simulink model "frbd_64ch_600mhz"  (R2013b)
settings: Solver=FixedStepDiscrete  SolverMode=SingleTasking  StartTime=0.0  StopTime=10.0  RelTol=1e-3
undefined symbols (not defined in the file or in its folder): pfb_coeff_gen_calc
libraries: xbsIndex_r4 x14695, casper_library_misc x59, casper_library_delays x32, dspsigops x16, casper_library_pfbs x2, xps_library x1
(part 24 of 145)

== system frbd_64ch_600mhz/Parallel_Dedispersor_v4/Dedispersor_v2_4 ==
  Data : Inport
  Valid : Inport  Port=2
  Counter : xbsIndex_r4/Counter  cnt_type=Free Running  cnt_to=Inf  operation=Up  start_count=0  cnt_by_val=1  arith_type=Unsigned  n_bits=4  bin_pt=0  load_pin=off  rst=off  en=on  explicit_period=on  period=1  dbl_ovrd=off  use_behavioral_HDL=off  implementation=Fabric  block_type=counter
  Mux : xbsIndex_r4/Mux  inputs=16  en=off  latency=0  precision=Full  arith_type=Unsigned  n_bits=16  bin_pt=14  quantization=Truncate  overflow=Wrap  dbl_ovrd=off  block_type=mux
  detector_block_v2 : Subsystem  AncestorBlock=honestlibrary/detector_block_v2  mask(Basic block for FRB detection){chn=0, lat=8, nbits=4}
      mask prompts: chn "Channel"; lat "Latency"; nbits "Number of Bits (Counter)"
      mask help:
      | Delays a certain channel a number of latency clock cycles, according to the fixed DM table.
      | This version incorporates an internal counter (nbits) to know when store or give a certain value.
      mask init:
      | detector_block_init_v2(gcb,'chn',chn,'lat',lat,'nbits',nbits)
      settings: AttributesFormatString=Channel: 0, Delay: 8
  detector_block_v21 : Subsystem  AncestorBlock=honestlibrary/detector_block_v2  mask(Basic block for FRB detection){chn=1, lat=20, nbits=4}
      mask prompts: chn "Channel"; lat "Latency"; nbits "Number of Bits (Counter)"
      mask help:
      | Delays a certain channel a number of latency clock cycles, according to the fixed DM table.
      | This version incorporates an internal counter (nbits) to know when store or give a certain value.
      mask init:
      | detector_block_init_v2(gcb,'chn',chn,'lat',lat,'nbits',nbits)
      settings: AttributesFormatString=Channel: 1, Delay: 20
  detector_block_v210 : Subsystem  AncestorBlock=honestlibrary/detector_block_v2  mask(Basic block for FRB detection){chn=10, lat=93, nbits=4}
      mask prompts: chn "Channel"; lat "Latency"; nbits "Number of Bits (Counter)"
      mask help:
      | Delays a certain channel a number of latency clock cycles, according to the fixed DM table.
      | This version incorporates an internal counter (nbits) to know when store or give a certain value.
      mask init:
      | detector_block_init_v2(gcb,'chn',chn,'lat',lat,'nbits',nbits)
      settings: AttributesFormatString=Channel: 10, Delay: 93
  detector_block_v211 : Subsystem  AncestorBlock=honestlibrary/detector_block_v2  mask(Basic block for FRB detection){chn=11, lat=99, nbits=4}
      mask prompts: chn "Channel"; lat "Latency"; nbits "Number of Bits (Counter)"
      mask help:
      | Delays a certain channel a number of latency clock cycles, according to the fixed DM table.
      | This version incorporates an internal counter (nbits) to know when store or give a certain value.
      mask init:
      | detector_block_init_v2(gcb,'chn',chn,'lat',lat,'nbits',nbits)
      settings: AttributesFormatString=Channel: 11, Delay: 99
  detector_block_v212 : Subsystem  AncestorBlock=honestlibrary/detector_block_v2  mask(Basic block for FRB detection){chn=12, lat=104, nbits=4}
      mask prompts: chn "Channel"; lat "Latency"; nbits "Number of Bits (Counter)"
      mask help:
      | Delays a certain channel a number of latency clock cycles, according to the fixed DM table.
      | This version incorporates an internal counter (nbits) to know when store or give a certain value.
      mask init:
      | detector_block_init_v2(gcb,'chn',chn,'lat',lat,'nbits',nbits)
      settings: AttributesFormatString=Channel: 12, Delay: 104
  detector_block_v213 : Subsystem  AncestorBlock=honestlibrary/detector_block_v2  mask(Basic block for FRB detection){chn=13, lat=108, nbits=4}
      mask prompts: chn "Channel"; lat "Latency"; nbits "Number of Bits (Counter)"
      mask help:
      | Delays a certain channel a number of latency clock cycles, according to the fixed DM table.
      | This version incorporates an internal counter (nbits) to know when store or give a certain value.
      mask init:
      | detector_block_init_v2(gcb,'chn',chn,'lat',lat,'nbits',nbits)
      settings: AttributesFormatString=Channel: 13, Delay: 108
  detector_block_v214 : Subsystem  AncestorBlock=honestlibrary/detector_block_v2  mask(Basic block for FRB detection){chn=14, lat=113, nbits=4}
      mask prompts: chn "Channel"; lat "Latency"; nbits "Number of Bits (Counter)"
      mask help:
      | Delays a certain channel a number of latency clock cycles, according to the fixed DM table.
      | This version incorporates an internal counter (nbits) to know when store or give a certain value.
      mask init:
      | detector_block_init_v2(gcb,'chn',chn,'lat',lat,'nbits',nbits)
      settings: AttributesFormatString=Channel: 14, Delay: 113
  detector_block_v215 : Subsystem  AncestorBlock=honestlibrary/detector_block_v2  mask(Basic block for FRB detection){chn=15, lat=117, nbits=4}
      mask prompts: chn "Channel"; lat "Latency"; nbits "Number of Bits (Counter)"
      mask help:
      | Delays a certain channel a number of latency clock cycles, according to the fixed DM table.
      | This version incorporates an internal counter (nbits) to know when store or give a certain value.
      mask init:
      | detector_block_init_v2(gcb,'chn',chn,'lat',lat,'nbits',nbits)
      settings: AttributesFormatString=Channel: 15, Delay: 117
  detector_block_v22 : Subsystem  AncestorBlock=honestlibrary/detector_block_v2  mask(Basic block for FRB detection){chn=2, lat=31, nbits=4}
      mask prompts: chn "Channel"; lat "Latency"; nbits "Number of Bits (Counter)"
      mask help:
      | Delays a certain channel a number of latency clock cycles, according to the fixed DM table.
      | This version incorporates an internal counter (nbits) to know when store or give a certain value.
      mask init:
      | detector_block_init_v2(gcb,'chn',chn,'lat',lat,'nbits',nbits)
      settings: AttributesFormatString=Channel: 2, Delay: 31
  detector_block_v23 : Subsystem  AncestorBlock=honestlibrary/detector_block_v2  mask(Basic block for FRB detection){chn=3, lat=41, nbits=4}
      mask prompts: chn "Channel"; lat "Latency"; nbits "Number of Bits (Counter)"
      mask help:
      | Delays a certain channel a number of latency clock cycles, according to the fixed DM table.
      | This version incorporates an internal counter (nbits) to know when store or give a certain value.
      mask init:
      | detector_block_init_v2(gcb,'chn',chn,'lat',lat,'nbits',nbits)
      settings: AttributesFormatString=Channel: 3, Delay: 41
  detector_block_v24 : Subsystem  AncestorBlock=honestlibrary/detector_block_v2  mask(Basic block for FRB detection){chn=4, lat=51, nbits=4}
      mask prompts: chn "Channel"; lat "Latency"; nbits "Number of Bits (Counter)"
      mask help:
      | Delays a certain channel a number of latency clock cycles, according to the fixed DM table.
      | This version incorporates an internal counter (nbits) to know when store or give a certain value.
      mask init:
      | detector_block_init_v2(gcb,'chn',chn,'lat',lat,'nbits',nbits)
      settings: AttributesFormatString=Channel: 4, Delay: 51
  detector_block_v25 : Subsystem  AncestorBlock=honestlibrary/detector_block_v2  mask(Basic block for FRB detection){chn=5, lat=59, nbits=4}
      mask prompts: chn "Channel"; lat "Latency"; nbits "Number of Bits (Counter)"
      mask help:
      | Delays a certain channel a number of latency clock cycles, according to the fixed DM table.
      | This version incorporates an internal counter (nbits) to know when store or give a certain value.
      mask init:
      | detector_block_init_v2(gcb,'chn',chn,'lat',lat,'nbits',nbits)
      settings: AttributesFormatString=Channel: 5, Delay: 59
  detector_block_v26 : Subsystem  AncestorBlock=honestlibrary/detector_block_v2  mask(Basic block for FRB detection){chn=6, lat=67, nbits=4}
      mask prompts: chn "Channel"; lat "Latency"; nbits "Number of Bits (Counter)"
      mask help:
      | Delays a certain channel a number of latency clock cycles, according to the fixed DM table.
      | This version incorporates an internal counter (nbits) to know when store or give a certain value.
      mask init:
      | detector_block_init_v2(gcb,'chn',chn,'lat',lat,'nbits',nbits)
      settings: AttributesFormatString=Channel: 6, Delay: 67
  detector_block_v27 : Subsystem  AncestorBlock=honestlibrary/detector_block_v2  mask(Basic block for FRB detection){chn=7, lat=74, nbits=4}
      mask prompts: chn "Channel"; lat "Latency"; nbits "Number of Bits (Counter)"
      mask help:
      | Delays a certain channel a number of latency clock cycles, according to the fixed DM table.
      | This version incorporates an internal counter (nbits) to know when store or give a certain value.
      mask init:
      | detector_block_init_v2(gcb,'chn',chn,'lat',lat,'nbits',nbits)
      settings: AttributesFormatString=Channel: 7, Delay: 74
  detector_block_v28 : Subsystem  AncestorBlock=honestlibrary/detector_block_v2  mask(Basic block for FRB detection){chn=8, lat=81, nbits=4}
      mask prompts: chn "Channel"; lat "Latency"; nbits "Number of Bits (Counter)"
      mask help:
      | Delays a certain channel a number of latency clock cycles, according to the fixed DM table.
      | This version incorporates an internal counter (nbits) to know when store or give a certain value.
      mask init:
      | detector_block_init_v2(gcb,'chn',chn,'lat',lat,'nbits',nbits)
      settings: AttributesFormatString=Channel: 8, Delay: 81
  detector_block_v29 : Subsystem  AncestorBlock=honestlibrary/detector_block_v2  mask(Basic block for FRB detection){chn=9, lat=87, nbits=4}
      mask prompts: chn "Channel"; lat "Latency"; nbits "Number of Bits (Counter)"
      mask help:
      | Delays a certain channel a number of latency clock cycles, according to the fixed DM table.
      | This version incorporates an internal counter (nbits) to know when store or give a certain value.
      mask init:
      | detector_block_init_v2(gcb,'chn',chn,'lat',lat,'nbits',nbits)
      settings: AttributesFormatString=Channel: 9, Delay: 87
  Output : Outport
  wires:
  Mux/1 -> Output/1
  detector_block_v215/1(Out1) -> Mux/17
  detector_block_v214/1(Out1) -> Mux/16
  detector_block_v213/1(Out1) -> Mux/15
  detector_block_v212/1(Out1) -> Mux/14
  detector_block_v211/1(Out1) -> Mux/13
  detector_block_v210/1(Out1) -> Mux/12
  detector_block_v29/1(Out1) -> Mux/11
  detector_block_v28/1(Out1) -> Mux/10
  detector_block_v27/1(Out1) -> Mux/9
  detector_block_v26/1(Out1) -> Mux/8
  detector_block_v25/1(Out1) -> Mux/7
  detector_block_v24/1(Out1) -> Mux/6
  detector_block_v23/1(Out1) -> Mux/5
  detector_block_v22/1(Out1) -> Mux/4
  detector_block_v21/1(Out1) -> Mux/3
  detector_block_v2/1(Out1) -> Mux/2
  Counter/1 -> Mux/1
  Valid/1 -> Counter/1, detector_block_v215/2(Valid), detector_block_v214/2(Valid), detector_block_v213/2(Valid), detector_block_v212/2(Valid), detector_block_v211/2(Valid), detector_block_v210/2(Valid), detector_block_v29/2(Valid), detector_block_v28/2(Valid), detector_block_v27/2(Valid), detector_block_v26/2(Valid), detector_block_v25/2(Valid), detector_block_v24/2(Valid), detector_block_v23/2(Valid), detector_block_v22/2(Valid), detector_block_v21/2(Valid), detector_block_v2/2(Valid)
  Data/1 -> detector_block_v215/1(Data), detector_block_v214/1(Data), detector_block_v213/1(Data), detector_block_v212/1(Data), detector_block_v211/1(Data), detector_block_v210/1(Data), detector_block_v29/1(Data), detector_block_v28/1(Data), detector_block_v27/1(Data), detector_block_v26/1(Data), detector_block_v25/1(Data), detector_block_v24/1(Data), detector_block_v23/1(Data), detector_block_v22/1(Data), detector_block_v21/1(Data), detector_block_v2/1(Data)

== system frbd_64ch_600mhz/Parallel_Dedispersor_v5/Dedispersor_v2_1 ==
  Data : Inport
  Valid : Inport  Port=2
  Counter : xbsIndex_r4/Counter  cnt_type=Free Running  cnt_to=Inf  operation=Up  start_count=0  cnt_by_val=1  arith_type=Unsigned  n_bits=4  bin_pt=0  load_pin=off  rst=off  en=on  explicit_period=on  period=1  dbl_ovrd=off  use_behavioral_HDL=off  implementation=Fabric  block_type=counter
  Mux : xbsIndex_r4/Mux  inputs=16  en=off  latency=0  precision=Full  arith_type=Unsigned  n_bits=16  bin_pt=14  quantization=Truncate  overflow=Wrap  dbl_ovrd=off  block_type=mux
  detector_block_v2 : Subsystem  AncestorBlock=honestlibrary/detector_block_v2  mask(Basic block for FRB detection){chn=0, lat=1, nbits=4}
      mask prompts: chn "Channel"; lat "Latency"; nbits "Number of Bits (Counter)"
      mask help:
      | Delays a certain channel a number of latency clock cycles, according to the fixed DM table.
      | This version incorporates an internal counter (nbits) to know when store or give a certain value.
      mask init:
      | detector_block_init_v2(gcb,'chn',chn,'lat',lat,'nbits',nbits)
      settings: AttributesFormatString=Channel: 0, Delay: 1
  detector_block_v21 : Subsystem  AncestorBlock=honestlibrary/detector_block_v2  mask(Basic block for FRB detection){chn=1, lat=12, nbits=4}
      mask prompts: chn "Channel"; lat "Latency"; nbits "Number of Bits (Counter)"
      mask help:
      | Delays a certain channel a number of latency clock cycles, according to the fixed DM table.
      | This version incorporates an internal counter (nbits) to know when store or give a certain value.
      mask init:
      | detector_block_init_v2(gcb,'chn',chn,'lat',lat,'nbits',nbits)
      settings: AttributesFormatString=Channel: 1, Delay: 12
  detector_block_v210 : Subsystem  AncestorBlock=honestlibrary/detector_block_v2  mask(Basic block for FRB detection){chn=10, lat=89, nbits=4}
      mask prompts: chn "Channel"; lat "Latency"; nbits "Number of Bits (Counter)"
      mask help:
      | Delays a certain channel a number of latency clock cycles, according to the fixed DM table.
      | This version incorporates an internal counter (nbits) to know when store or give a certain value.
      mask init:
      | detector_block_init_v2(gcb,'chn',chn,'lat',lat,'nbits',nbits)
      settings: AttributesFormatString=Channel: 10, Delay: 89
  detector_block_v211 : Subsystem  AncestorBlock=honestlibrary/detector_block_v2  mask(Basic block for FRB detection){chn=11, lat=95, nbits=4}
      mask prompts: chn "Channel"; lat "Latency"; nbits "Number of Bits (Counter)"
      mask help:
      | Delays a certain channel a number of latency clock cycles, according to the fixed DM table.
      | This version incorporates an internal counter (nbits) to know when store or give a certain value.
      mask init:
      | detector_block_init_v2(gcb,'chn',chn,'lat',lat,'nbits',nbits)
      settings: AttributesFormatString=Channel: 11, Delay: 95
  detector_block_v212 : Subsystem  AncestorBlock=honestlibrary/detector_block_v2  mask(Basic block for FRB detection){chn=12, lat=100, nbits=4}
      mask prompts: chn "Channel"; lat "Latency"; nbits "Number of Bits (Counter)"
      mask help:
      | Delays a certain channel a number of latency clock cycles, according to the fixed DM table.
      | This version incorporates an internal counter (nbits) to know when store or give a certain value.
      mask init:
      | detector_block_init_v2(gcb,'chn',chn,'lat',lat,'nbits',nbits)
      settings: AttributesFormatString=Channel: 12, Delay: 100
  detector_block_v213 : Subsystem  AncestorBlock=honestlibrary/detector_block_v2  mask(Basic block for FRB detection){chn=13, lat=105, nbits=4}
      mask prompts: chn "Channel"; lat "Latency"; nbits "Number of Bits (Counter)"
      mask help:
      | Delays a certain channel a number of latency clock cycles, according to the fixed DM table.
      | This version incorporates an internal counter (nbits) to know when store or give a certain value.
      mask init:
      | detector_block_init_v2(gcb,'chn',chn,'lat',lat,'nbits',nbits)
      settings: AttributesFormatString=Channel: 13, Delay: 105
  detector_block_v214 : Subsystem  AncestorBlock=honestlibrary/detector_block_v2  mask(Basic block for FRB detection){chn=14, lat=110, nbits=4}
      mask prompts: chn "Channel"; lat "Latency"; nbits "Number of Bits (Counter)"
      mask help:
      | Delays a certain channel a number of latency clock cycles, according to the fixed DM table.
      | This version incorporates an internal counter (nbits) to know when store or give a certain value.
      mask init:
      | detector_block_init_v2(gcb,'chn',chn,'lat',lat,'nbits',nbits)
      settings: AttributesFormatString=Channel: 14, Delay: 110
  detector_block_v215 : Subsystem  AncestorBlock=honestlibrary/detector_block_v2  mask(Basic block for FRB detection){chn=15, lat=114, nbits=4}
      mask prompts: chn "Channel"; lat "Latency"; nbits "Number of Bits (Counter)"
      mask help:
      | Delays a certain channel a number of latency clock cycles, according to the fixed DM table.
      | This version incorporates an internal counter (nbits) to know when store or give a certain value.
      mask init:
      | detector_block_init_v2(gcb,'chn',chn,'lat',lat,'nbits',nbits)
      settings: AttributesFormatString=Channel: 15, Delay: 114
  detector_block_v22 : Subsystem  AncestorBlock=honestlibrary/detector_block_v2  mask(Basic block for FRB detection){chn=2, lat=23, nbits=4}
      mask prompts: chn "Channel"; lat "Latency"; nbits "Number of Bits (Counter)"
      mask help:
      | Delays a certain channel a number of latency clock cycles, according to the fixed DM table.
      | This version incorporates an internal counter (nbits) to know when store or give a certain value.
      mask init:
      | detector_block_init_v2(gcb,'chn',chn,'lat',lat,'nbits',nbits)
      settings: AttributesFormatString=Channel: 2, Delay: 23
  detector_block_v23 : Subsystem  AncestorBlock=honestlibrary/detector_block_v2  mask(Basic block for FRB detection){chn=3, lat=34, nbits=4}
      mask prompts: chn "Channel"; lat "Latency"; nbits "Number of Bits (Counter)"
      mask help:
      | Delays a certain channel a number of latency clock cycles, according to the fixed DM table.
      | This version incorporates an internal counter (nbits) to know when store or give a certain value.
      mask init:
      | detector_block_init_v2(gcb,'chn',chn,'lat',lat,'nbits',nbits)
      settings: AttributesFormatString=Channel: 3, Delay: 34
  detector_block_v24 : Subsystem  AncestorBlock=honestlibrary/detector_block_v2  mask(Basic block for FRB detection){chn=4, lat=44, nbits=4}
      mask prompts: chn "Channel"; lat "Latency"; nbits "Number of Bits (Counter)"
      mask help:
      | Delays a certain channel a number of latency clock cycles, according to the fixed DM table.
      | This version incorporates an internal counter (nbits) to know when store or give a certain value.
      mask init:
      | detector_block_init_v2(gcb,'chn',chn,'lat',lat,'nbits',nbits)
      settings: AttributesFormatString=Channel: 4, Delay: 44
  detector_block_v25 : Subsystem  AncestorBlock=honestlibrary/detector_block_v2  mask(Basic block for FRB detection){chn=5, lat=53, nbits=4}
      mask prompts: chn "Channel"; lat "Latency"; nbits "Number of Bits (Counter)"
      mask help:
      | Delays a certain channel a number of latency clock cycles, according to the fixed DM table.
      | This version incorporates an internal counter (nbits) to know when store or give a certain value.
      mask init:
      | detector_block_init_v2(gcb,'chn',chn,'lat',lat,'nbits',nbits)
      settings: AttributesFormatString=Channel: 5, Delay: 53
  detector_block_v26 : Subsystem  AncestorBlock=honestlibrary/detector_block_v2  mask(Basic block for FRB detection){chn=6, lat=61, nbits=4}
      mask prompts: chn "Channel"; lat "Latency"; nbits "Number of Bits (Counter)"
      mask help:
      | Delays a certain channel a number of latency clock cycles, according to the fixed DM table.
      | This version incorporates an internal counter (nbits) to know when store or give a certain value.
      mask init:
      | detector_block_init_v2(gcb,'chn',chn,'lat',lat,'nbits',nbits)
      settings: AttributesFormatString=Channel: 6, Delay: 61
  detector_block_v27 : Subsystem  AncestorBlock=honestlibrary/detector_block_v2  mask(Basic block for FRB detection){chn=7, lat=69, nbits=4}
      mask prompts: chn "Channel"; lat "Latency"; nbits "Number of Bits (Counter)"
      mask help:
      | Delays a certain channel a number of latency clock cycles, according to the fixed DM table.
      | This version incorporates an internal counter (nbits) to know when store or give a certain value.
      mask init:
      | detector_block_init_v2(gcb,'chn',chn,'lat',lat,'nbits',nbits)
      settings: AttributesFormatString=Channel: 7, Delay: 69
  detector_block_v28 : Subsystem  AncestorBlock=honestlibrary/detector_block_v2  mask(Basic block for FRB detection){chn=8, lat=76, nbits=4}
      mask prompts: chn "Channel"; lat "Latency"; nbits "Number of Bits (Counter)"
      mask help:
      | Delays a certain channel a number of latency clock cycles, according to the fixed DM table.
      | This version incorporates an internal counter (nbits) to know when store or give a certain value.
      mask init:
      | detector_block_init_v2(gcb,'chn',chn,'lat',lat,'nbits',nbits)
      settings: AttributesFormatString=Channel: 8, Delay: 76
  detector_block_v29 : Subsystem  AncestorBlock=honestlibrary/detector_block_v2  mask(Basic block for FRB detection){chn=9, lat=83, nbits=4}
      mask prompts: chn "Channel"; lat "Latency"; nbits "Number of Bits (Counter)"
      mask help:
      | Delays a certain channel a number of latency clock cycles, according to the fixed DM table.
      | This version incorporates an internal counter (nbits) to know when store or give a certain value.
      mask init:
      | detector_block_init_v2(gcb,'chn',chn,'lat',lat,'nbits',nbits)
      settings: AttributesFormatString=Channel: 9, Delay: 83
  Output : Outport
  wires:
  Data/1 -> detector_block_v2/1(Data), detector_block_v21/1(Data), detector_block_v22/1(Data), detector_block_v23/1(Data), detector_block_v24/1(Data), detector_block_v25/1(Data), detector_block_v26/1(Data), detector_block_v27/1(Data), detector_block_v28/1(Data), detector_block_v29/1(Data), detector_block_v210/1(Data), detector_block_v211/1(Data), detector_block_v212/1(Data), detector_block_v213/1(Data), detector_block_v214/1(Data), detector_block_v215/1(Data)
  Valid/1 -> detector_block_v2/2(Valid), detector_block_v21/2(Valid), detector_block_v22/2(Valid), detector_block_v23/2(Valid), detector_block_v24/2(Valid), detector_block_v25/2(Valid), detector_block_v26/2(Valid), detector_block_v27/2(Valid), detector_block_v28/2(Valid), detector_block_v29/2(Valid), detector_block_v210/2(Valid), detector_block_v211/2(Valid), detector_block_v212/2(Valid), detector_block_v213/2(Valid), detector_block_v214/2(Valid), detector_block_v215/2(Valid), Counter/1
  Counter/1 -> Mux/1
  detector_block_v2/1(Out1) -> Mux/2
  detector_block_v21/1(Out1) -> Mux/3
  detector_block_v22/1(Out1) -> Mux/4
  detector_block_v23/1(Out1) -> Mux/5
  detector_block_v24/1(Out1) -> Mux/6
  detector_block_v25/1(Out1) -> Mux/7
  detector_block_v26/1(Out1) -> Mux/8
  detector_block_v27/1(Out1) -> Mux/9
  detector_block_v28/1(Out1) -> Mux/10
  detector_block_v29/1(Out1) -> Mux/11
  detector_block_v210/1(Out1) -> Mux/12
  detector_block_v211/1(Out1) -> Mux/13
  detector_block_v212/1(Out1) -> Mux/14
  detector_block_v213/1(Out1) -> Mux/15
  detector_block_v214/1(Out1) -> Mux/16
  detector_block_v215/1(Out1) -> Mux/17
  Mux/1 -> Output/1

== system frbd_64ch_600mhz/Parallel_Dedispersor_v5/Dedispersor_v2_2 ==
  Data : Inport
  Valid : Inport  Port=2
  Counter : xbsIndex_r4/Counter  cnt_type=Free Running  cnt_to=Inf  operation=Up  start_count=0  cnt_by_val=1  arith_type=Unsigned  n_bits=4  bin_pt=0  load_pin=off  rst=off  en=on  explicit_period=on  period=1  dbl_ovrd=off  use_behavioral_HDL=off  implementation=Fabric  block_type=counter
  Mux : xbsIndex_r4/Mux  inputs=16  en=off  latency=0  precision=Full  arith_type=Unsigned  n_bits=16  bin_pt=14  quantization=Truncate  overflow=Wrap  dbl_ovrd=off  block_type=mux
  detector_block_v2 : Subsystem  AncestorBlock=honestlibrary/detector_block_v2  mask(Basic block for FRB detection){chn=0, lat=2, nbits=4}
      mask prompts: chn "Channel"; lat "Latency"; nbits "Number of Bits (Counter)"
      mask help:
      | Delays a certain channel a number of latency clock cycles, according to the fixed DM table.
      | This version incorporates an internal counter (nbits) to know when store or give a certain value.
      mask init:
      | detector_block_init_v2(gcb,'chn',chn,'lat',lat,'nbits',nbits)
      settings: AttributesFormatString=Channel: 0, Delay: 2
  detector_block_v21 : Subsystem  AncestorBlock=honestlibrary/detector_block_v2  mask(Basic block for FRB detection){chn=1, lat=15, nbits=4}
      mask prompts: chn "Channel"; lat "Latency"; nbits "Number of Bits (Counter)"
      mask help:
      | Delays a certain channel a number of latency clock cycles, according to the fixed DM table.
      | This version incorporates an internal counter (nbits) to know when store or give a certain value.
      mask init:
      | detector_block_init_v2(gcb,'chn',chn,'lat',lat,'nbits',nbits)
      settings: AttributesFormatString=Channel: 1, Delay: 15
  detector_block_v210 : Subsystem  AncestorBlock=honestlibrary/detector_block_v2  mask(Basic block for FRB detection){chn=10, lat=90, nbits=4}
      mask prompts: chn "Channel"; lat "Latency"; nbits "Number of Bits (Counter)"
      mask help:
      | Delays a certain channel a number of latency clock cycles, according to the fixed DM table.
      | This version incorporates an internal counter (nbits) to know when store or give a certain value.
      mask init:
      | detector_block_init_v2(gcb,'chn',chn,'lat',lat,'nbits',nbits)
      settings: AttributesFormatString=Channel: 10, Delay: 90
  detector_block_v211 : Subsystem  AncestorBlock=honestlibrary/detector_block_v2  mask(Basic block for FRB detection){chn=11, lat=96, nbits=4}
      mask prompts: chn "Channel"; lat "Latency"; nbits "Number of Bits (Counter)"
      mask help:
      | Delays a certain channel a number of latency clock cycles, according to the fixed DM table.
      | This version incorporates an internal counter (nbits) to know when store or give a certain value.
      mask init:
      | detector_block_init_v2(gcb,'chn',chn,'lat',lat,'nbits',nbits)
      settings: AttributesFormatString=Channel: 11, Delay: 96
  detector_block_v212 : Subsystem  AncestorBlock=honestlibrary/detector_block_v2  mask(Basic block for FRB detection){chn=12, lat=101, nbits=4}
      mask prompts: chn "Channel"; lat "Latency"; nbits "Number of Bits (Counter)"
      mask help:
      | Delays a certain channel a number of latency clock cycles, according to the fixed DM table.
      | This version incorporates an internal counter (nbits) to know when store or give a certain value.
      mask init:
      | detector_block_init_v2(gcb,'chn',chn,'lat',lat,'nbits',nbits)
      settings: AttributesFormatString=Channel: 12, Delay: 101
  detector_block_v213 : Subsystem  AncestorBlock=honestlibrary/detector_block_v2  mask(Basic block for FRB detection){chn=13, lat=106, nbits=4}
      mask prompts: chn "Channel"; lat "Latency"; nbits "Number of Bits (Counter)"
      mask help:
      | Delays a certain channel a number of latency clock cycles, according to the fixed DM table.
      | This version incorporates an internal counter (nbits) to know when store or give a certain value.
      mask init:
      | detector_block_init_v2(gcb,'chn',chn,'lat',lat,'nbits',nbits)
      settings: AttributesFormatString=Channel: 13, Delay: 106
  detector_block_v214 : Subsystem  AncestorBlock=honestlibrary/detector_block_v2  mask(Basic block for FRB detection){chn=14, lat=111, nbits=4}
      mask prompts: chn "Channel"; lat "Latency"; nbits "Number of Bits (Counter)"
      mask help:
      | Delays a certain channel a number of latency clock cycles, according to the fixed DM table.
      | This version incorporates an internal counter (nbits) to know when store or give a certain value.
      mask init:
      | detector_block_init_v2(gcb,'chn',chn,'lat',lat,'nbits',nbits)
      settings: AttributesFormatString=Channel: 14, Delay: 111
  detector_block_v215 : Subsystem  AncestorBlock=honestlibrary/detector_block_v2  mask(Basic block for FRB detection){chn=15, lat=115, nbits=4}
      mask prompts: chn "Channel"; lat "Latency"; nbits "Number of Bits (Counter)"
      mask help:
      | Delays a certain channel a number of latency clock cycles, according to the fixed DM table.
      | This version incorporates an internal counter (nbits) to know when store or give a certain value.
      mask init:
      | detector_block_init_v2(gcb,'chn',chn,'lat',lat,'nbits',nbits)
      settings: AttributesFormatString=Channel: 15, Delay: 115
  detector_block_v22 : Subsystem  AncestorBlock=honestlibrary/detector_block_v2  mask(Basic block for FRB detection){chn=2, lat=26, nbits=4}
      mask prompts: chn "Channel"; lat "Latency"; nbits "Number of Bits (Counter)"
      mask help:
      | Delays a certain channel a number of latency clock cycles, according to the fixed DM table.
      | This version incorporates an internal counter (nbits) to know when store or give a certain value.
      mask init:
      | detector_block_init_v2(gcb,'chn',chn,'lat',lat,'nbits',nbits)
      settings: AttributesFormatString=Channel: 2, Delay: 26
  detector_block_v23 : Subsystem  AncestorBlock=honestlibrary/detector_block_v2  mask(Basic block for FRB detection){chn=3, lat=37, nbits=4}
      mask prompts: chn "Channel"; lat "Latency"; nbits "Number of Bits (Counter)"
      mask help:
      | Delays a certain channel a number of latency clock cycles, according to the fixed DM table.
      | This version incorporates an internal counter (nbits) to know when store or give a certain value.
      mask init:
      | detector_block_init_v2(gcb,'chn',chn,'lat',lat,'nbits',nbits)
      settings: AttributesFormatString=Channel: 3, Delay: 37
  detector_block_v24 : Subsystem  AncestorBlock=honestlibrary/detector_block_v2  mask(Basic block for FRB detection){chn=4, lat=46, nbits=4}
      mask prompts: chn "Channel"; lat "Latency"; nbits "Number of Bits (Counter)"
      mask help:
      | Delays a certain channel a number of latency clock cycles, according to the fixed DM table.
      | This version incorporates an internal counter (nbits) to know when store or give a certain value.
      mask init:
      | detector_block_init_v2(gcb,'chn',chn,'lat',lat,'nbits',nbits)
      settings: AttributesFormatString=Channel: 4, Delay: 46
  detector_block_v25 : Subsystem  AncestorBlock=honestlibrary/detector_block_v2  mask(Basic block for FRB detection){chn=5, lat=55, nbits=4}
      mask prompts: chn "Channel"; lat "Latency"; nbits "Number of Bits (Counter)"
      mask help:
      | Delays a certain channel a number of latency clock cycles, according to the fixed DM table.
      | This version incorporates an internal counter (nbits) to know when store or give a certain value.
      mask init:
      | detector_block_init_v2(gcb,'chn',chn,'lat',lat,'nbits',nbits)
      settings: AttributesFormatString=Channel: 5, Delay: 55
  detector_block_v26 : Subsystem  AncestorBlock=honestlibrary/detector_block_v2  mask(Basic block for FRB detection){chn=6, lat=63, nbits=4}
      mask prompts: chn "Channel"; lat "Latency"; nbits "Number of Bits (Counter)"
      mask help:
      | Delays a certain channel a number of latency clock cycles, according to the fixed DM table.
      | This version incorporates an internal counter (nbits) to know when store or give a certain value.
      mask init:
      | detector_block_init_v2(gcb,'chn',chn,'lat',lat,'nbits',nbits)
      settings: AttributesFormatString=Channel: 6, Delay: 63
  detector_block_v27 : Subsystem  AncestorBlock=honestlibrary/detector_block_v2  mask(Basic block for FRB detection){chn=7, lat=71, nbits=4}
      mask prompts: chn "Channel"; lat "Latency"; nbits "Number of Bits (Counter)"
      mask help:
      | Delays a certain channel a number of latency clock cycles, according to the fixed DM table.
      | This version incorporates an internal counter (nbits) to know when store or give a certain value.
      mask init:
      | detector_block_init_v2(gcb,'chn',chn,'lat',lat,'nbits',nbits)
      settings: AttributesFormatString=Channel: 7, Delay: 71
  detector_block_v28 : Subsystem  AncestorBlock=honestlibrary/detector_block_v2  mask(Basic block for FRB detection){chn=8, lat=78, nbits=4}
      mask prompts: chn "Channel"; lat "Latency"; nbits "Number of Bits (Counter)"
      mask help:
      | Delays a certain channel a number of latency clock cycles, according to the fixed DM table.
      | This version incorporates an internal counter (nbits) to know when store or give a certain value.
      mask init:
      | detector_block_init_v2(gcb,'chn',chn,'lat',lat,'nbits',nbits)
      settings: AttributesFormatString=Channel: 8, Delay: 78
  detector_block_v29 : Subsystem  AncestorBlock=honestlibrary/detector_block_v2  mask(Basic block for FRB detection){chn=9, lat=84, nbits=4}
      mask prompts: chn "Channel"; lat "Latency"; nbits "Number of Bits (Counter)"
      mask help:
      | Delays a certain channel a number of latency clock cycles, according to the fixed DM table.
      | This version incorporates an internal counter (nbits) to know when store or give a certain value.
      mask init:
      | detector_block_init_v2(gcb,'chn',chn,'lat',lat,'nbits',nbits)
      settings: AttributesFormatString=Channel: 9, Delay: 84
  Output : Outport
  wires:
  Data/1 -> detector_block_v2/1(Data), detector_block_v21/1(Data), detector_block_v22/1(Data), detector_block_v23/1(Data), detector_block_v24/1(Data), detector_block_v25/1(Data), detector_block_v26/1(Data), detector_block_v27/1(Data), detector_block_v28/1(Data), detector_block_v29/1(Data), detector_block_v210/1(Data), detector_block_v211/1(Data), detector_block_v212/1(Data), detector_block_v213/1(Data), detector_block_v214/1(Data), detector_block_v215/1(Data)
  Valid/1 -> detector_block_v2/2(Valid), detector_block_v21/2(Valid), detector_block_v22/2(Valid), detector_block_v23/2(Valid), detector_block_v24/2(Valid), detector_block_v25/2(Valid), detector_block_v26/2(Valid), detector_block_v27/2(Valid), detector_block_v28/2(Valid), detector_block_v29/2(Valid), detector_block_v210/2(Valid), detector_block_v211/2(Valid), detector_block_v212/2(Valid), detector_block_v213/2(Valid), detector_block_v214/2(Valid), detector_block_v215/2(Valid), Counter/1
  Counter/1 -> Mux/1
  detector_block_v2/1(Out1) -> Mux/2
  detector_block_v21/1(Out1) -> Mux/3
  detector_block_v22/1(Out1) -> Mux/4
  detector_block_v23/1(Out1) -> Mux/5
  detector_block_v24/1(Out1) -> Mux/6
  detector_block_v25/1(Out1) -> Mux/7
  detector_block_v26/1(Out1) -> Mux/8
  detector_block_v27/1(Out1) -> Mux/9
  detector_block_v28/1(Out1) -> Mux/10
  detector_block_v29/1(Out1) -> Mux/11
  detector_block_v210/1(Out1) -> Mux/12
  detector_block_v211/1(Out1) -> Mux/13
  detector_block_v212/1(Out1) -> Mux/14
  detector_block_v213/1(Out1) -> Mux/15
  detector_block_v214/1(Out1) -> Mux/16
  detector_block_v215/1(Out1) -> Mux/17
  Mux/1 -> Output/1

== system frbd_64ch_600mhz/Parallel_Dedispersor_v5/Dedispersor_v2_3 ==
  Data : Inport
  Valid : Inport  Port=2
  Counter : xbsIndex_r4/Counter  cnt_type=Free Running  cnt_to=Inf  operation=Up  start_count=0  cnt_by_val=1  arith_type=Unsigned  n_bits=4  bin_pt=0  load_pin=off  rst=off  en=on  explicit_period=on  period=1  dbl_ovrd=off  use_behavioral_HDL=off  implementation=Fabric  block_type=counter
  Mux : xbsIndex_r4/Mux  inputs=16  en=off  latency=0  precision=Full  arith_type=Unsigned  n_bits=16  bin_pt=14  quantization=Truncate  overflow=Wrap  dbl_ovrd=off  block_type=mux
  detector_block_v2 : Subsystem  AncestorBlock=honestlibrary/detector_block_v2  mask(Basic block for FRB detection){chn=0, lat=5, nbits=4}
      mask prompts: chn "Channel"; lat "Latency"; nbits "Number of Bits (Counter)"
      mask help:
      | Delays a certain channel a number of latency clock cycles, according to the fixed DM table.
      | This version incorporates an internal counter (nbits) to know when store or give a certain value.
      mask init:
      | detector_block_init_v2(gcb,'chn',chn,'lat',lat,'nbits',nbits)
      settings: AttributesFormatString=Channel: 0, Delay: 5
  detector_block_v21 : Subsystem  AncestorBlock=honestlibrary/detector_block_v2  mask(Basic block for FRB detection){chn=1, lat=18, nbits=4}
      mask prompts: chn "Channel"; lat "Latency"; nbits "Number of Bits (Counter)"
      mask help:
      | Delays a certain channel a number of latency clock cycles, according to the fixed DM table.
      | This version incorporates an internal counter (nbits) to know when store or give a certain value.
      mask init:
      | detector_block_init_v2(gcb,'chn',chn,'lat',lat,'nbits',nbits)
      settings: AttributesFormatString=Channel: 1, Delay: 18
  detector_block_v210 : Subsystem  AncestorBlock=honestlibrary/detector_block_v2  mask(Basic block for FRB detection){chn=10, lat=92, nbits=4}
      mask prompts: chn "Channel"; lat "Latency"; nbits "Number of Bits (Counter)"
      mask help:
      | Delays a certain channel a number of latency clock cycles, according to the fixed DM table.
      | This version incorporates an internal counter (nbits) to know when store or give a certain value.
      mask init:
      | detector_block_init_v2(gcb,'chn',chn,'lat',lat,'nbits',nbits)
      settings: AttributesFormatString=Channel: 10, Delay: 92
  detector_block_v211 : Subsystem  AncestorBlock=honestlibrary/detector_block_v2  mask(Basic block for FRB detection){chn=11, lat=97, nbits=4}
      mask prompts: chn "Channel"; lat "Latency"; nbits "Number of Bits (Counter)"
      mask help:
      | Delays a certain channel a number of latency clock cycles, according to the fixed DM table.
      | This version incorporates an internal counter (nbits) to know when store or give a certain value.
      mask init:
      | detector_block_init_v2(gcb,'chn',chn,'lat',lat,'nbits',nbits)
      settings: AttributesFormatString=Channel: 11, Delay: 97
  detector_block_v212 : Subsystem  AncestorBlock=honestlibrary/detector_block_v2  mask(Basic block for FRB detection){chn=12, lat=102, nbits=4}
      mask prompts: chn "Channel"; lat "Latency"; nbits "Number of Bits (Counter)"
      mask help:
      | Delays a certain channel a number of latency clock cycles, according to the fixed DM table.
      | This version incorporates an internal counter (nbits) to know when store or give a certain value.
      mask init:
      | detector_block_init_v2(gcb,'chn',chn,'lat',lat,'nbits',nbits)
      settings: AttributesFormatString=Channel: 12, Delay: 102
  detector_block_v213 : Subsystem  AncestorBlock=honestlibrary/detector_block_v2  mask(Basic block for FRB detection){chn=13, lat=107, nbits=4}
      mask prompts: chn "Channel"; lat "Latency"; nbits "Number of Bits (Counter)"
      mask help:
      | Delays a certain channel a number of latency clock cycles, according to the fixed DM table.
      | This version incorporates an internal counter (nbits) to know when store or give a certain value.
      mask init:
      | detector_block_init_v2(gcb,'chn',chn,'lat',lat,'nbits',nbits)
      settings: AttributesFormatString=Channel: 13, Delay: 107
  detector_block_v214 : Subsystem  AncestorBlock=honestlibrary/detector_block_v2  mask(Basic block for FRB detection){chn=14, lat=112, nbits=4}
      mask prompts: chn "Channel"; lat "Latency"; nbits "Number of Bits (Counter)"
      mask help:
      | Delays a certain channel a number of latency clock cycles, according to the fixed DM table.
      | This version incorporates an internal counter (nbits) to know when store or give a certain value.
      mask init:
      | detector_block_init_v2(gcb,'chn',chn,'lat',lat,'nbits',nbits)
      settings: AttributesFormatString=Channel: 14, Delay: 112
  detector_block_v215 : Subsystem  AncestorBlock=honestlibrary/detector_block_v2  mask(Basic block for FRB detection){chn=15, lat=116, nbits=4}
      mask prompts: chn "Channel"; lat "Latency"; nbits "Number of Bits (Counter)"
      mask help:
      | Delays a certain channel a number of latency clock cycles, according to the fixed DM table.
      | This version incorporates an internal counter (nbits) to know when store or give a certain value.
      mask init:
      | detector_block_init_v2(gcb,'chn',chn,'lat',lat,'nbits',nbits)
      settings: AttributesFormatString=Channel: 15, Delay: 116
  detector_block_v22 : Subsystem  AncestorBlock=honestlibrary/detector_block_v2  mask(Basic block for FRB detection){chn=2, lat=29, nbits=4}
      mask prompts: chn "Channel"; lat "Latency"; nbits "Number of Bits (Counter)"
      mask help:
      | Delays a certain channel a number of latency clock cycles, according to the fixed DM table.
      | This version incorporates an internal counter (nbits) to know when store or give a certain value.
      mask init:
      | detector_block_init_v2(gcb,'chn',chn,'lat',lat,'nbits',nbits)
      settings: AttributesFormatString=Channel: 2, Delay: 29
  detector_block_v23 : Subsystem  AncestorBlock=honestlibrary/detector_block_v2  mask(Basic block for FRB detection){chn=3, lat=39, nbits=4}
      mask prompts: chn "Channel"; lat "Latency"; nbits "Number of Bits (Counter)"
      mask help:
      | Delays a certain channel a number of latency clock cycles, according to the fixed DM table.
      | This version incorporates an internal counter (nbits) to know when store or give a certain value.
      mask init:
      | detector_block_init_v2(gcb,'chn',chn,'lat',lat,'nbits',nbits)
      settings: AttributesFormatString=Channel: 3, Delay: 39
  detector_block_v24 : Subsystem  AncestorBlock=honestlibrary/detector_block_v2  mask(Basic block for FRB detection){chn=4, lat=48, nbits=4}
      mask prompts: chn "Channel"; lat "Latency"; nbits "Number of Bits (Counter)"
      mask help:
      | Delays a certain channel a number of latency clock cycles, according to the fixed DM table.
      | This version incorporates an internal counter (nbits) to know when store or give a certain value.
      mask init:
      | detector_block_init_v2(gcb,'chn',chn,'lat',lat,'nbits',nbits)
      settings: AttributesFormatString=Channel: 4, Delay: 48
  detector_block_v25 : Subsystem  AncestorBlock=honestlibrary/detector_block_v2  mask(Basic block for FRB detection){chn=5, lat=57, nbits=4}
      mask prompts: chn "Channel"; lat "Latency"; nbits "Number of Bits (Counter)"
      mask help:
      | Delays a certain channel a number of latency clock cycles, according to the fixed DM table.
      | This version incorporates an internal counter (nbits) to know when store or give a certain value.
      mask init:
      | detector_block_init_v2(gcb,'chn',chn,'lat',lat,'nbits',nbits)
      settings: AttributesFormatString=Channel: 5, Delay: 57
  detector_block_v26 : Subsystem  AncestorBlock=honestlibrary/detector_block_v2  mask(Basic block for FRB detection){chn=6, lat=65, nbits=4}
      mask prompts: chn "Channel"; lat "Latency"; nbits "Number of Bits (Counter)"
      mask help:
      | Delays a certain channel a number of latency clock cycles, according to the fixed DM table.
      | This version incorporates an internal counter (nbits) to know when store or give a certain value.
      mask init:
      | detector_block_init_v2(gcb,'chn',chn,'lat',lat,'nbits',nbits)
      settings: AttributesFormatString=Channel: 6, Delay: 65
  detector_block_v27 : Subsystem  AncestorBlock=honestlibrary/detector_block_v2  mask(Basic block for FRB detection){chn=7, lat=73, nbits=4}
      mask prompts: chn "Channel"; lat "Latency"; nbits "Number of Bits (Counter)"
      mask help:
      | Delays a certain channel a number of latency clock cycles, according to the fixed DM table.
      | This version incorporates an internal counter (nbits) to know when store or give a certain value.
      mask init:
      | detector_block_init_v2(gcb,'chn',chn,'lat',lat,'nbits',nbits)
      settings: AttributesFormatString=Channel: 7, Delay: 73
  detector_block_v28 : Subsystem  AncestorBlock=honestlibrary/detector_block_v2  mask(Basic block for FRB detection){chn=8, lat=79, nbits=4}
      mask prompts: chn "Channel"; lat "Latency"; nbits "Number of Bits (Counter)"
      mask help:
      | Delays a certain channel a number of latency clock cycles, according to the fixed DM table.
      | This version incorporates an internal counter (nbits) to know when store or give a certain value.
      mask init:
      | detector_block_init_v2(gcb,'chn',chn,'lat',lat,'nbits',nbits)
      settings: AttributesFormatString=Channel: 8, Delay: 79
  detector_block_v29 : Subsystem  AncestorBlock=honestlibrary/detector_block_v2  mask(Basic block for FRB detection){chn=9, lat=86, nbits=4}
      mask prompts: chn "Channel"; lat "Latency"; nbits "Number of Bits (Counter)"
      mask help:
      | Delays a certain channel a number of latency clock cycles, according to the fixed DM table.
      | This version incorporates an internal counter (nbits) to know when store or give a certain value.
      mask init:
      | detector_block_init_v2(gcb,'chn',chn,'lat',lat,'nbits',nbits)
      settings: AttributesFormatString=Channel: 9, Delay: 86
  Output : Outport
  wires:
  Data/1 -> detector_block_v2/1(Data), detector_block_v21/1(Data), detector_block_v22/1(Data), detector_block_v23/1(Data), detector_block_v24/1(Data), detector_block_v25/1(Data), detector_block_v26/1(Data), detector_block_v27/1(Data), detector_block_v28/1(Data), detector_block_v29/1(Data), detector_block_v210/1(Data), detector_block_v211/1(Data), detector_block_v212/1(Data), detector_block_v213/1(Data), detector_block_v214/1(Data), detector_block_v215/1(Data)
  Valid/1 -> detector_block_v2/2(Valid), detector_block_v21/2(Valid), detector_block_v22/2(Valid), detector_block_v23/2(Valid), detector_block_v24/2(Valid), detector_block_v25/2(Valid), detector_block_v26/2(Valid), detector_block_v27/2(Valid), detector_block_v28/2(Valid), detector_block_v29/2(Valid), detector_block_v210/2(Valid), detector_block_v211/2(Valid), detector_block_v212/2(Valid), detector_block_v213/2(Valid), detector_block_v214/2(Valid), detector_block_v215/2(Valid), Counter/1
  Counter/1 -> Mux/1
  detector_block_v2/1(Out1) -> Mux/2
  detector_block_v21/1(Out1) -> Mux/3
  detector_block_v22/1(Out1) -> Mux/4
  detector_block_v23/1(Out1) -> Mux/5
  detector_block_v24/1(Out1) -> Mux/6
  detector_block_v25/1(Out1) -> Mux/7
  detector_block_v26/1(Out1) -> Mux/8
  detector_block_v27/1(Out1) -> Mux/9
  detector_block_v28/1(Out1) -> Mux/10
  detector_block_v29/1(Out1) -> Mux/11
  detector_block_v210/1(Out1) -> Mux/12
  detector_block_v211/1(Out1) -> Mux/13
  detector_block_v212/1(Out1) -> Mux/14
  detector_block_v213/1(Out1) -> Mux/15
  detector_block_v214/1(Out1) -> Mux/16
  detector_block_v215/1(Out1) -> Mux/17
  Mux/1 -> Output/1
